simulink model "assignment_2_g"  (R2020a)
settings: Solver=VariableStepAuto  StartTime=0.0  StopTime=30  RelTol=1e-3
settings Model: Creator=David Wiman  LastModifiedBy=David Wiman

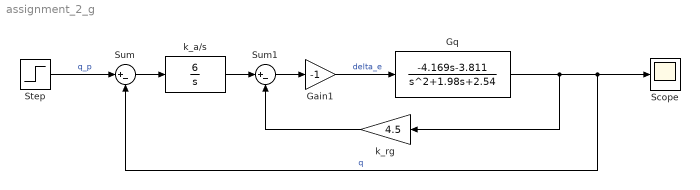
== system assignment_2_g ==
  Gain1 : Gain  Gain=-1
  Gq : TransferFcn  Numerator=[-4.169 -3.811]  Denominator=[1 1.98 2.54]
  Scope : Scope
  Step : Step  SampleTime=0
  Sum : Sum  Inputs=|+-
  Sum1 : Sum  Inputs=|+-
  k_a/s : TransferFcn  Numerator=[6]  Denominator=[1 0]
  k_rg : Gain  Gain=4.5
  wires:
  Step/1 -> Sum/1  "q_p"
  Sum/1 -> k_a/s/1
  k_a/s/1 -> Sum1/1
  Sum1/1 -> Gain1/1
  Gain1/1 -> Gq/1  "delta_e"
  Gq/1 -> Scope/1, Sum/2, k_rg/1  "q"
  k_rg/1 -> Sum1/2
